simulink model "velocity_control_model"  (R2021a)
settings: Solver=FixedStepAuto  StartTime=0.0  StopTime=2.0  FixedStep=0.01  RelTol=1e-3
undefined symbols (not defined in the file or in its folder): Kd, Ki, Kp
settings Model: Creator=elissaito  LastModifiedBy=elissaito

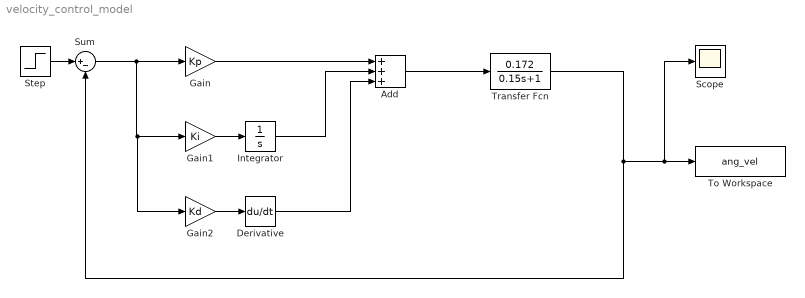
== system velocity_control_model ==
  Add : Sum  Inputs=+++
  Derivative : Derivative
  Gain : Gain  Gain=Kp
  Gain1 : Gain  Gain=Ki
  Gain2 : Gain  Gain=Kd
  Integrator : Integrator
  Scope : Scope
  Step : Step  Time=0  After=15  SampleTime=0
  Sum : Sum  Inputs=|+-
  To Workspace : ToWorkspace  VariableName=ang_vel  SaveFormat=Timeseries  SampleTime=-1
  Transfer Fcn : TransferFcn  Numerator=[0.172]  Denominator=[0.15 1]
  wires:
  Gain2/1 -> Derivative/1
  Gain1/1 -> Integrator/1
  Sum/1 -> Gain2/1, Gain1/1, Gain/1
  Gain/1 -> Add/1
  Integrator/1 -> Add/2
  Derivative/1 -> Add/3
  Add/1 -> Transfer Fcn/1
  Transfer Fcn/1 -> Scope/1, To Workspace/1, Sum/2
  Step/1 -> Sum/1
